simulink model "conventional_PID"  (R2024a)
settings: Solver=VariableStepAuto  StartTime=0.0  StopTime=10.0  RelTol=1e-3
settings Model: Creator=Miko  LastModifiedBy=Miko

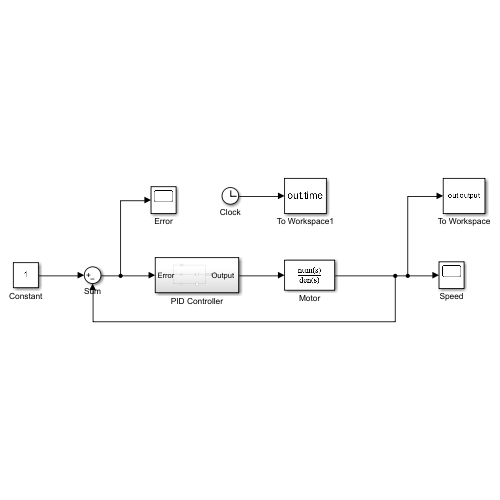
[thumbnail: Simulink's stored preview of the top-level diagram]
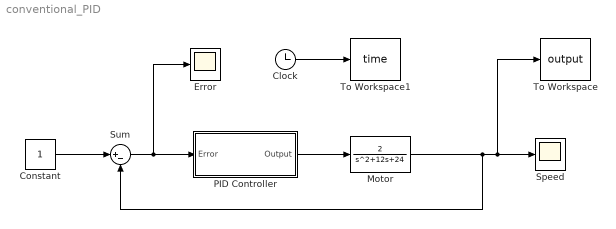
== system conventional_PID ==
  Clock : Clock
  Constant : Constant
  Error : Scope
  Motor : TransferFcn  Numerator=[2]  Denominator=[1 12 24]
  PID Controller : Subsystem
  Speed : Scope
  Sum : Sum  Inputs=|+-
  To Workspace : ToWorkspace  VariableName=output  SampleTime=-1
      settings: Save2DSignal=2-D array (concatenate along first dimension)
  To Workspace1 : ToWorkspace  VariableName=time  SampleTime=-1
      settings: Save2DSignal=2-D array (concatenate along first dimension)
  wires:
  Constant/1 -> Sum/1
  Sum/1 -> PID Controller/1(Error), Error/1
  Clock/1 -> To Workspace1/1
  PID Controller/1("Output ") -> Motor/1
  Motor/1 -> Sum/2, To Workspace/1, Speed/1

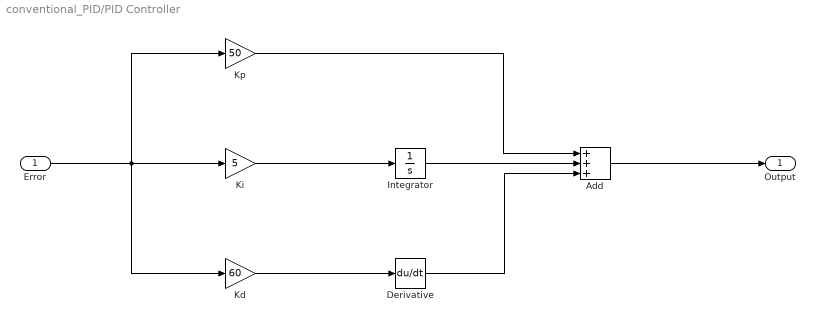
== system conventional_PID/PID Controller ==
  Error : Inport
  Add : Sum  Inputs=+++
  Derivative : Derivative
  Integrator : Integrator
  Kd : Gain  Gain=60
  Ki : Gain  Gain=5
  Kp : Gain  Gain=50
  "Output " : Outport
  wires:
  Error/1 -> Kd/1, Kp/1, Ki/1
  Ki/1 -> Integrator/1
  Kd/1 -> Derivative/1
  Integrator/1 -> Add/2
  Add/1 -> "Output "/1
  Kp/1 -> Add/1
  Derivative/1 -> Add/3
